simulink model "MSP_mt_test"  (R2016b)
settings: Solver=FixedStepAuto  StartTime=0.0  StopTime=20  FixedStep=0.001  RelTol=1e-3
settings Model: Creator=evich  LastModifiedBy=evich

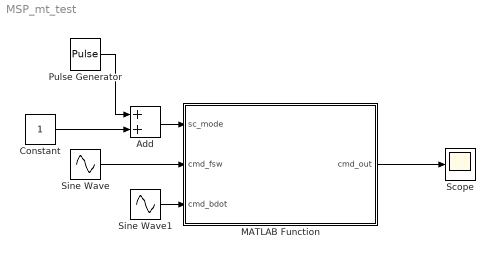
== system MSP_mt_test ==
  Add : Sum
  Constant : Constant
  MATLAB Function : MATLAB Function  TreatAsAtomicUnit=on
  Pulse Generator : DiscretePulseGenerator  PulseType=Time based  Period=5  PulseWidth=50
  Scope : Scope
  Sine Wave : Sin  SampleTime=0
  Sine Wave1 : Sin  Amplitude=7  Frequency=4  SampleTime=0
  wires:
  Sine Wave/1 -> MATLAB Function/2(cmd_fsw)
  Sine Wave1/1 -> MATLAB Function/3(cmd_bdot)
  MATLAB Function/1(cmd_out) -> Scope/1
  Constant/1 -> Add/2
  Add/1 -> MATLAB Function/1(sc_mode)
  Pulse Generator/1 -> Add/1

== matlab function MSP_mt_test/MATLAB Function ==
  data: sc_mode input; cmd_out output; cmd_fsw input; cmd_bdot input
function cmd_out = MT_logic(sc_mode,cmd_fsw,cmd_bdot)

% Chooses which control signal to pass through based on the sc_mode
%   mode_logic.bdot             = 1;
%   mode_logic.desat_eclipse    = 2;
%   mode_logic.point            = 3;
%       point.velocity          = 31;
%       point.ground            = 32;
%       point.MPC               = 33;
%   mode_logic.low_power        = 4;

% Note: If sc_mode = 0, then ADCS FSW is assumed to be powered off and the
% bdot command will automatically be passed through

if( sc_mode == 0 ) % ADCS FSW is powered off
    cmd_out = cmd_bdot;
else
    if( sc_mode == 1 ) % ADCS FSW indicates a tumble
        cmd_out = cmd_bdot;
    else
        cmd_out = cmd_fsw; % ADCS FSW wants control
    end
end
